simulink model "prac_pid"  (R2020a)
settings: Solver=VariableStepAuto  StartTime=0.0  StopTime=100  RelTol=1e-3
model workspace (MAT data in the model file):
  n = Simulink.Parameter
  n.Value = 1000000
  n.DataType = 'auto'
  n.Dimensions = [1 1]
settings Model: Creator=kishan  LastModifiedBy=kishan
settings SolverCC: ZeroCrossAlgorithm=Adaptive  AlgebraicLoopSolver=LineSearch
settings DebuggingCC: IgnoredZcDiagnostic=none

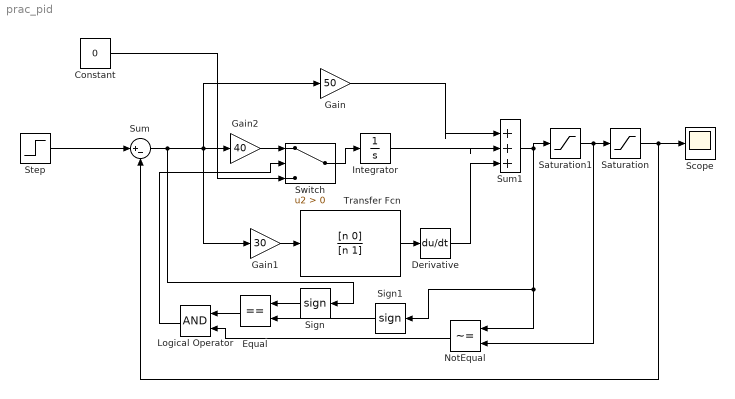
== system prac_pid ==
  Constant : Constant  Value=0
  Derivative : Derivative
  Equal : RelationalOperator  Operator===  OutDataTypeStr=boolean  RndMeth=Simplest
  Gain : Gain  Gain=50
  Gain1 : Gain  Gain=30
  Gain2 : Gain  Gain=40
  Integrator : Integrator
  Logical Operator : Logic  AllPortsSameDT=off  OutDataTypeStr=boolean
  NotEqual : RelationalOperator  Operator=~=  OutDataTypeStr=boolean  RndMeth=Simplest
  Saturation : Saturate  UpperLimit=75  LowerLimit=-75
  Saturation1 : Saturate  UpperLimit=50  LowerLimit=-50
  Scope : Scope
  Sign : Signum
  Sign1 : Signum
  Step : Step  After=100  SampleTime=0  ZeroCross=off
  Sum : Sum  Inputs=|+-
  Sum1 : Sum  Inputs=|+++
  Switch : Switch  Criteria=u2 > Threshold
  Transfer Fcn : TransferFcn  Numerator=[n 0]  Denominator=[n 1]
  wires:
  Sum/1 -> Sign/1, Gain2/1, Gain/1, Gain1/1
  Integrator/1 -> Sum1/2
  Gain/1 -> Sum1/1
  Derivative/1 -> Sum1/3
  Saturation/1 -> Sum/2, Scope/1
  Step/1 -> Sum/1
  Gain1/1 -> Transfer Fcn/1
  Transfer Fcn/1 -> Derivative/1
  Switch/1 -> Integrator/1
  Saturation1/1 -> NotEqual/2, Saturation/1
  Sum1/1 -> Saturation1/1, Sign1/1, NotEqual/1
  Gain2/1 -> Switch/1
  Constant/1 -> Switch/3
  Equal/1 -> Logical Operator/1
  NotEqual/1 -> Logical Operator/2
  Logical Operator/1 -> Switch/2
  Sign/1 -> Equal/1
  Sign1/1 -> Equal/2
